simulink model "sensorExpoler1_1"  (R2026a)
settings: Solver=FixedStepDiscrete  StopTime=inf  FixedStep=0.001
StopFcn:
  | plot_and_save_schmitt
undefined symbols (not defined in the file): Blocking, Non
libraries: amg_usbconverter_n_connect_lib x2
settings Model: Creator=pboon  LastModifiedBy=Itthiphat

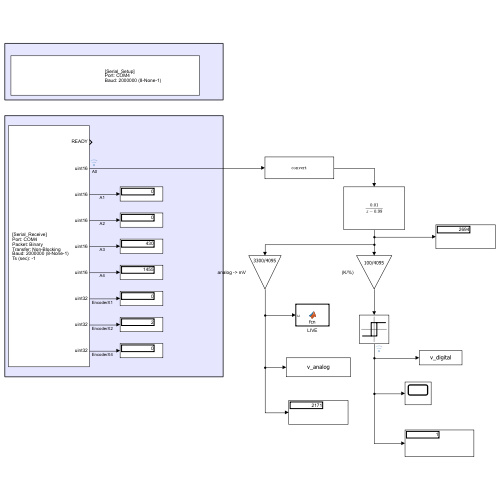
[thumbnail: Simulink's stored preview of the top-level diagram]
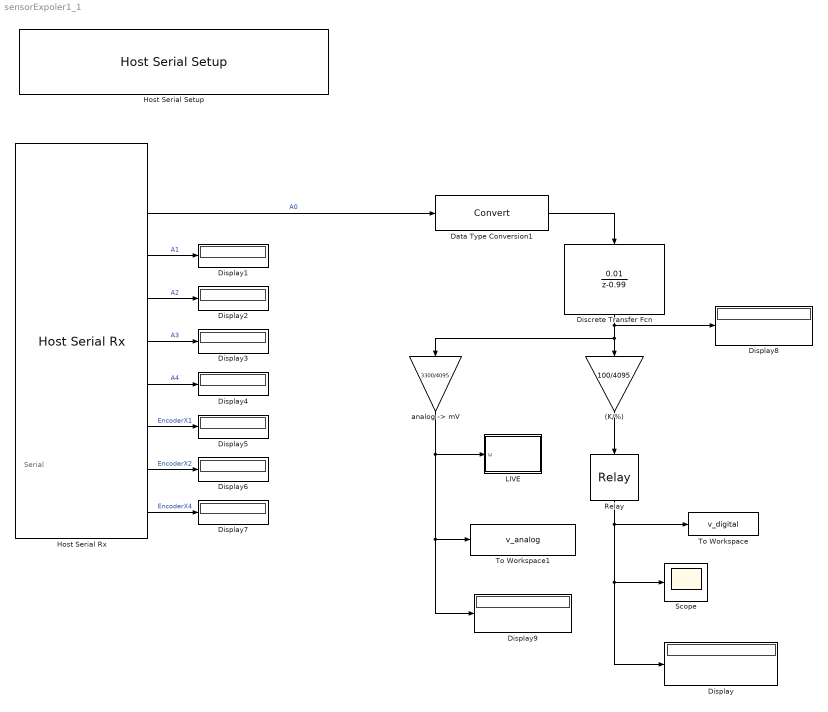
== system sensorExpoler1_1 ==
  note: Serial
  (K/%) : Gain  Gain=100/4095
  Data Type Conversion1 : DataTypeConversion  SaturateOnIntegerOverflow=off  RndMeth=Floor
  Discrete Transfer Fcn : DiscreteTransferFcn  Numerator=[0.01]  Denominator=[1 -0.99]
  Display{,1..9} (10 alike) : Display
  Host Serial Rx : amg_usbconverter_n_connect_lib/Host Serial Rx  conf=rx  port=<auto>  baudrate=2000000  databits=8  parity=None  stopbit=1  flowcontrol=None  transfer=Non-Blocking  timeout=5  packetmode=Binary  enableinitialvalues=off  initialvalues=[]  binheader='25'  binterminator='4E 4E'  porttype_double=0  porttype_single=0  porttype_int8=0  porttype_uint8=0  porttype_int16=0  porttype_uint16=5  porttype_int32=0  porttype_uint32=3  asciiformat='%d,%f'  rx_asciiterminator="CRLF (0x0D 0x0A - \"\\r\\n\")"  tx_asciiterminator="CRLF (0x0D 0x0A - \"\\r\\n\")"  sampletime=0.001  enablecustomportlabel=off  cinputportlabel=0  coutputportlabel=A  portpinstr=0  blockid=HostSerialRx  inputporttype=[]  inputportwidth=[]  inputportlabel={}  outputporttype=[3 5 5 5 5 5 7 7 7]  outputportwidth=[1 1 1 1 1 1 1 1 1]  outputportlabel={'READY','uint16','uint16','uint16','uint16','uint16','uint32','uint32','uint32'}  compat=0  optionstring=[]  autoport='COM4'
  Host Serial Setup : amg_usbconverter_n_connect_lib/Host Serial Setup  conf=setup  port=<auto>  baudrate=2000000  databits=8  parity=None  stopbit=1  flowcontrol=None  transfer=Blocking  timeout=2  packetmode=Binary  initialvalues=[]  binheader='7E 7E'  binterminator='03 03'  porttype_double=0  porttype_single=1  porttype_int8=0  porttype_uint8=0  porttype_int16=0  porttype_uint16=0  porttype_int32=0  porttype_uint32=2  asciiformat='%d %u %x'  rx_asciiterminator="CRLF (0x0D 0x0A - \"\\r\\n\")"  tx_asciiterminator="CRLF (0x0D 0x0A - \"\\r\\n\")"  sampletime=-1  enablecustomportlabel=off  cinputportlabel=0  coutputportlabel=A  portpinstr=0  blockid=HostSerialSetup  inputporttype=[]  inputportwidth=[]  inputportlabel={}  outputporttype=[]  outputportwidth=[]  outputportlabel={}  compat=0  optionstring=[]  autoport='COM4'
  LIVE : MATLAB Function  TreatAsAtomicUnit=on
  Relay : Relay  OnSwitchValue=60  OffSwitchValue=40
  Scope : Scope
  To Workspace : ToWorkspace  VariableName=v_digital  SaveFormat=Timeseries  SampleTime=-1
  To Workspace1 : ToWorkspace  VariableName=v_analog  SaveFormat=Timeseries  SampleTime=-1
  "analog -> mV" : Gain  Gain=3300/4095
  wires:
  Host Serial Rx/3 -> Display1/1  "A1"
  Host Serial Rx/4 -> Display2/1  "A2"
  Host Serial Rx/5 -> Display3/1  "A3"
  Host Serial Rx/6 -> Display4/1  "A4"
  Host Serial Rx/7 -> Display5/1  "EncoderX1"
  Host Serial Rx/8 -> Display6/1  "EncoderX2"
  Host Serial Rx/9 -> Display7/1  "EncoderX4"
  Host Serial Rx/2 -> Data Type Conversion1/1  "A0"
  Data Type Conversion1/1 -> Discrete Transfer Fcn/1
  Discrete Transfer Fcn/1 -> (K/%)/1, "analog -> mV"/1, Display8/1
  (K/%)/1 -> Relay/1
  Relay/1 -> To Workspace/1, Scope/1, Display/1
  "analog -> mV"/1 -> LIVE/1(u), To Workspace1/1, Display9/1

== matlab function sensorExpoler1_1/LIVE ==
  data: u input
function fcn(u)
    coder.extrinsic('assignin');
    assignin('base', 'live_v', u);
end
